simulink model "Target"  (R2023a)
settings: Solver=VariableStepAuto  StartTime=0.0  StopTime=10.0  RelTol=1e-3
settings Model: Creator=aan18022  LastModifiedBy=asd19005

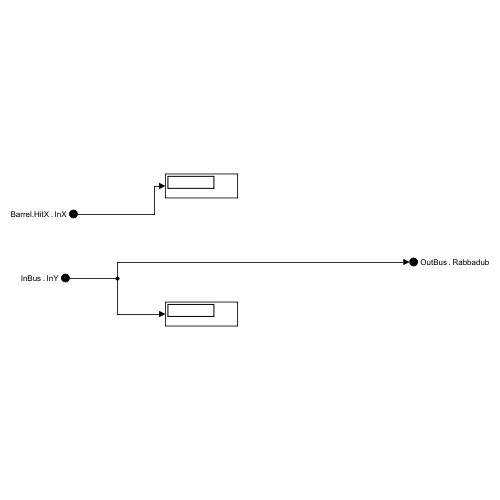
[thumbnail: Simulink's stored preview of the top-level diagram]
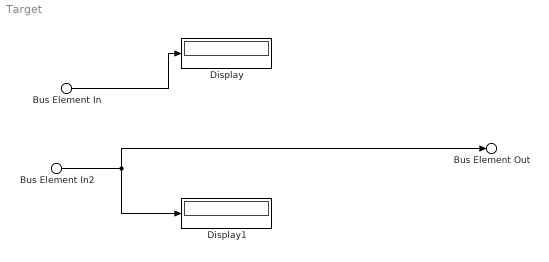
== system Target ==
  Bus Element In : Inport  PortName=Barrel.HitX  Element=InX
  Bus Element In2 : Inport  Port=2  PortName=Barrel.HitY  Element=InY
  Display : Display
  Display1 : Display
  Bus Element Out : Outport  PortName=OutBus  Element=Rabbadub
  wires:
  Bus Element In/1 -> Display/1
  Bus Element In2/1 -> Bus Element Out/1, Display1/1
